simulink model "ProyectoControl"  (R2020b)
settings: Solver=VariableStepAuto  StartTime=0.0  StopTime=25  RelTol=1e-3
values from neighbouring files (symbols this model uses):
  A = [-0.0558 0.08 -0.997 0.0415 0.0033 ... (first row only)    [Control_proyecto.m]
  B = [0 0.00729 ... (first row only)    [Control_proyecto.m]
  C = [0 0 0 1 0 ... (first row only)    [Control_proyecto.m]
  D = [0 0;0 0]    [Control_proyecto.m]
  Ki = [Kaug(:,6) Kaug(:,7)]    [Control_proyecto.m]
  Kp = Kaug(:,1:5)    [Control_proyecto.m]
  lambda = 0.5    [Control_proyecto.m]
undefined symbols (not defined in the file or in its folder): DiscIntNeverNeededParam, L, sigbuilder_block
libraries: simulink_extras x10, simulink x3, eeGeneralControl x1
settings Model: Creator=agustin  LastModifiedBy=agustin

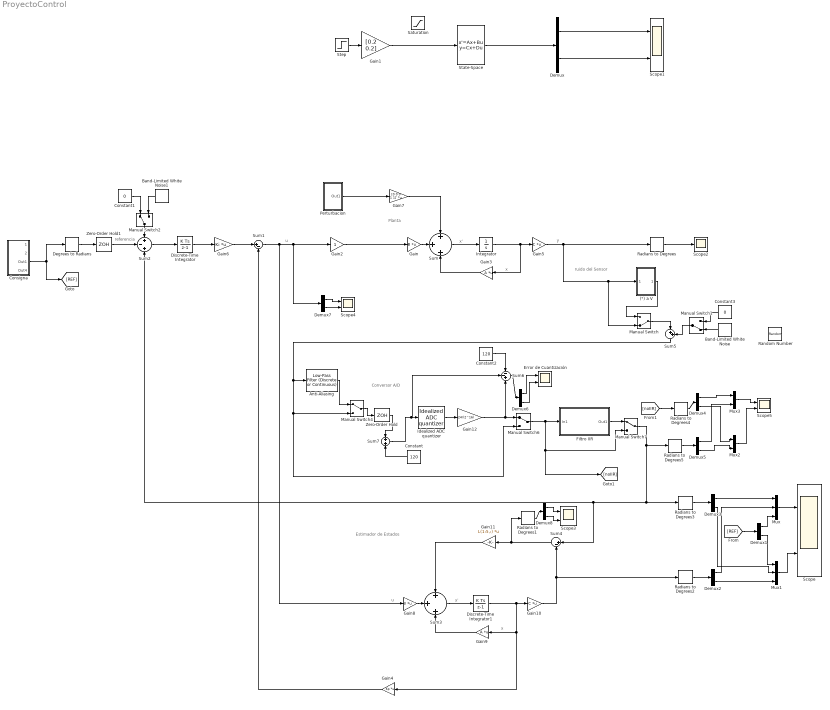
== system ProyectoControl ==
  note: Conversor A/D
  note: ruido del Sensor
  note: Estimador de Estados
  note: referencia
  note: Planta
  note: y
  note: x
  note: x'
  note: u
  note: x
  note: x'
  note: u
  (°) a V : Subsystem
  Anti-Aliasing : eeGeneralControl/Low-Pass Filter (Discrete or Continuous)  K=1  T=0.01  B=inf  A=-inf  init_option=Inherited from block input  x0=0  Ts=-1
  Band-Limited White Noise : simulink/Sources/Band-Limited White Noise  Cov=[70e-9]  Ts=0.1  seed=[23341]
  Band-Limited White Noise1 : simulink/Sources/Band-Limited White Noise  Cov=[0.25e-6]  Ts=0.1  seed=[23341]
  Consigna : Subsystem
  Constant : Constant  Value=120
  Constant1 : Constant  Value=0
  Constant2 : Constant  Value=120
  Constant3 : Constant  Value=0
  Degrees to Radians : simulink_extras/Transformations/Degrees to Radians
  Demux{,1..8} (9 alike) : Demux  Outputs=2
  Discrete-Time Integrator : DiscreteIntegrator  SampleTime=-1  ICPrevOutput=DiscIntNeverNeededParam  ICPrevScaledInput=DiscIntNeverNeededParam
  Discrete-Time Integrator1 : DiscreteIntegrator  SampleTime=-1  ICPrevOutput=DiscIntNeverNeededParam  ICPrevScaledInput=DiscIntNeverNeededParam
  Error de Cuantización : Scope  NumInputPorts=2
  Filtro IIR : Subsystem
  Gain : Gain  Gain=B  Multiplication=Matrix(K*u)
  Gain1 : Gain  Gain=[0.2 0.2]
  Gain10 : Gain  Gain=C  Multiplication=Matrix(K*u)
  Gain11 : Gain  Gain=L(1:5,:)  Multiplication=Matrix(K*u)
  Gain12 : Gain  Gain=24/(2^16)
  Gain2 : Gain
  Gain3 : Gain  Gain=A  Multiplication=Matrix(K*u)
  Gain4 : Gain  Gain=Kp  Multiplication=Matrix(K*u)
  Gain5 : Gain  Gain=C  Multiplication=Matrix(K*u)
  Gain6 : Gain  Gain=Ki  Multiplication=Matrix(K*u)
  Gain7 : Gain  Gain=[0 0 0 1 1]'  Multiplication=Matrix(K*u)
  Gain8 : Gain  Gain=B  Multiplication=Matrix(K*u)
  Gain9 : Gain  Gain=A  Multiplication=Matrix(K*u)
  Idealized ADC quantizer : simulink_extras/Additional Discrete/Idealized ADC quantizer  NumberOfConverterBits=16  Vmin=100  Vmax=140  OutputDataType=int32  OutputNegativeValues=on
  Integrator : Integrator
  Manual Switch : ManualSwitch  CurrentSetting=0
  Manual Switch1 : ManualSwitch  CurrentSetting=0
  Manual Switch{2,4,6..7} (4 alike) : ManualSwitch
  Mux : Mux  Inputs=3
  Mux1 : Mux  Inputs=3
  Mux2 : Mux  Inputs=2
  Mux3 : Mux  Inputs=2
  Perturbacion : Subsystem
  Radians to Degrees{,1..5} (6 alike) : simulink_extras/Transformations/Radians to Degrees
  Random Number : RandomNumber  Variance=70e-9  SampleTime=0.1
  Saturation : Saturate  UpperLimit=1  LowerLimit=-1
  Scope{,1,3..5} (5 alike) : Scope  NumInputPorts=2
  Scope2 : Scope
  State-Space : StateSpace  A=A  B=B  C=C  D=D  InitialCondition=0  ContinuousStateAttributes='position'
  Step : Step  SampleTime=0
  Sum : Sum  Inputs=+|+|+
  Sum1 : Sum  Inputs=|+-
  Sum2 : Sum  Inputs=+-+
  Sum3 : Sum  Inputs=+|+|+
  Sum4 : Sum  Inputs=|+-
  Sum5 : Sum  Inputs=|++
  Sum6 : Sum  Inputs=--+
  Sum7 : Sum
  Zero-Order Hold : ZeroOrderHold  SampleTime=1e-3
  Zero-Order Hold1 : ZeroOrderHold  SampleTime=1e-3
  wires:
  State-Space/1 -> Demux/1
  Step/1 -> Gain1/1
  Demux/1 -> Scope1/1
  Demux/2 -> Scope1/2
  Gain1/1 -> State-Space/1
  Gain/1 -> Sum/2
  Gain3/1 -> Sum/3
  Sum/1 -> Integrator/1
  Integrator/1 -> Gain3/1, Gain5/1
  Gain4/1 -> Sum1/2
  Gain6/1 -> Sum1/1
  Sum2/1 -> Discrete-Time Integrator/1
  Gain7/1 -> Sum/1
  Discrete-Time Integrator/1 -> Gain6/1
  Gain11/1 -> Sum3/1
  Gain8/1 -> Sum3/2
  Sum3/1 -> Discrete-Time Integrator1/1
  Gain9/1 -> Sum3/3
  Discrete-Time Integrator1/1 -> Gain4/1, Gain9/1, Gain10/1
  Sum1/1 -> Demux7/1, Gain2/1, Gain8/1
  Gain10/1 -> Sum4/2, Radians to Degrees2/1
  Sum4/1 -> Gain11/1, Radians to Degrees1/1
  Sum5/1 -> Anti-Aliasing/1, Manual Switch4/2, Manual Switch6/2
  Constant3/1 -> Manual Switch1/1
  Manual Switch1/1 -> Sum5/2
  Zero-Order Hold/1 -> Sum7/1
  Idealized ADC quantizer/1 -> Gain12/1
  Gain12/1 -> Sum6/3, Manual Switch6/1
  Filtro IIR/1(Out1) -> Manual Switch7/1
  Radians to Degrees1/1 -> Demux8/1
  Radians to Degrees2/1 -> Demux2/1
  Manual Switch4/1 -> Zero-Order Hold/1
  Anti-Aliasing/1 -> Manual Switch4/1
  Manual Switch6/1 -> Filtro IIR/1(In1), [noIIR], Manual Switch7/2
  Manual Switch7/1 -> Radians to Degrees5/1, Sum2/3, Sum4/1, Radians to Degrees3/1
  Zero-Order Hold1/1 -> Sum2/2
  Degrees to Radians/1 -> Zero-Order Hold1/1
  [REF] -> Demux1/1
  Perturbacion/1(Out1) -> Gain7/1
  Band-Limited White Noise1/1 -> Manual Switch2/2
  Constant1/1 -> Manual Switch2/1
  Manual Switch2/1 -> Sum2/1
  Consigna/3(Out1) -> [REF], Degrees to Radians/1
  Mux/1 -> Scope/1
  Mux1/1 -> Scope/2
  Radians to Degrees3/1 -> Demux3/1
  Demux2/2 -> Mux1/3
  Demux2/1 -> Mux/2
  Demux3/2 -> Mux1/2
  Demux1/2 -> Mux1/1
  Demux3/1 -> Mux/1
  Demux1/1 -> Mux/3
  [noIIR] -> Radians to Degrees4/1
  Mux3/1 -> Scope5/1
  Mux2/1 -> Scope5/2
  Demux4/1 -> Mux3/1
  Demux5/1 -> Mux3/2
  Demux4/2 -> Mux2/1
  Demux5/2 -> Mux2/2
  Radians to Degrees4/1 -> Demux4/1
  Radians to Degrees5/1 -> Demux5/1
  Sum6/1 -> Demux6/1
  Demux6/1 -> Error de Cuantización/1
  Demux6/2 -> Error de Cuantización/2
  Demux7/1 -> Scope4/1
  Demux7/2 -> Scope4/2
  Gain2/1 -> Gain/1
  Demux8/1 -> Scope3/1
  Demux8/2 -> Scope3/2
  Band-Limited White Noise/1 -> Manual Switch1/2
  Constant/1 -> Sum7/2
  Sum7/1 -> Sum6/2, Idealized ADC quantizer/1
  Constant2/1 -> Sum6/1
  Gain5/1 -> Radians to Degrees/1, Manual Switch/2, (°) a V/1(In1)
  Radians to Degrees/1 -> Scope2/1
  (°) a V/1(Out1) -> Manual Switch/1
  Manual Switch/1 -> Sum5/1

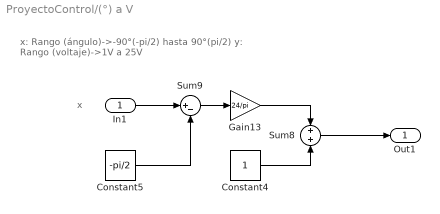
== system ProyectoControl/(°) a V ==
  note: x
  note: x: Rango (ángulo)->-90°(-pi/2) hasta 90°(pi/2)
      | y: Rango (voltaje)->1V a 25V
  In1 : Inport
  Constant4 : Constant
  Constant5 : Constant  Value=-pi/2
  Gain13 : Gain  Gain=24/pi
  Sum8 : Sum
  Sum9 : Sum  Inputs=|+-
  Out1 : Outport
  wires:
  In1/1 -> Sum9/1
  Constant5/1 -> Sum9/2
  Sum9/1 -> Gain13/1
  Sum8/1 -> Out1/1
  Gain13/1 -> Sum8/1
  Constant4/1 -> Sum8/2

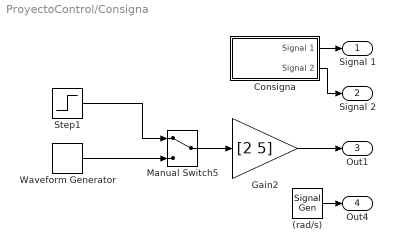
== system ProyectoControl/Consigna ==
  "(rad/s) " : SignalGenerator  WaveForm=square  Amplitude=0.2  Frequency=0.1  Units=rad/sec
  Consigna : Subsystem  Tag=STV Subsys  LoadFcn=sigbuilder_block('load');  StartFcn=sigbuilder_block('start');  StopFcn=sigbuilder_block('stop');  ClipboardFcn=sigbuilder_block('clipboard');  mask(Sigbuilder block){tuvar=[0:10]}
      mask help: Simulink:masks:SigbuilderBlock_MD
      mask init:
      | if ~strcmp(get_param(bdroot(gcbh),'SimulationStatus'),'stopped') tuvar = sigbuilder_block('maskInit'); end
      settings: CopyFcn=sigbuilder_block('copy');  DeleteFcn=sigbuilder_block('delete');  ModelCloseFcn=sigbuilder_block('modelClose');  PreSaveFcn=sigbuilder_block('preSave');  PauseFcn=sigbuilder_block('pause');  ContinueFcn=sigbuilder_block('continue');  NameChangeFcn=sigbuilder_block('namechange');  OpenFcn=sigbuilder_block('open',[311.25 87.75 550.5 359.25 ]);  CloseFcn=sigbuilder_block('close');
      mask Display: plot(0, 0, 100, 100,[2, 2, 32, 32, 2], [68, 8, 8, 68, 68],[32, 2], [38, 38], [32, 19, 2],[53, 60, 44], [32, 17, 17, 2],[16, 16, 31, 31]);txt = getActiveGroup(gcbh);text(2, 100, txt,'verticalAlignment', 'top');
  Gain2 : Gain  Gain=[2 5]
  Manual Switch5 : ManualSwitch
  Step1 : Step  SampleTime=0
  Waveform Generator : simulink/Sources/Waveform Generator  OutMin=[]  OutMax=[]  OutDataTypeStr=double  SelectedSignal=1  Signals=sin('Amplitude', 1, 'Frequency', 0.1, 'Phase', 0)  BlockNames=MultiportSwitch_92f0ff05a9a94f3  SampleTime=0.1
  Signal 1 : Outport
  Signal 2 : Outport  Port=2
  Out1 : Outport  Port=3
  Out4 : Outport  Port=4
  wires:
  Gain2/1 -> Out1/1
  Manual Switch5/1 -> Gain2/1
  Step1/1 -> Manual Switch5/1
  Waveform Generator/1 -> Manual Switch5/2
  "(rad/s) "/1 -> Out4/1
  Consigna/1(Signal 1) -> Signal 1/1
  Consigna/2(Signal 2) -> Signal 2/1

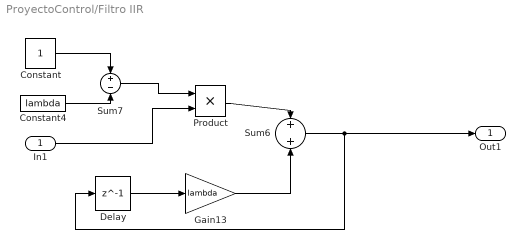
== system ProyectoControl/Filtro IIR ==
  In1 : Inport
  Constant : Constant
  Constant4 : Constant  Value=lambda
  Delay : Delay  DelayLength=1  InitialCondition=0
  Gain13 : Gain  Gain=lambda
  Product : Product
  Sum6 : Sum
  Sum7 : Sum  Inputs=+-
  Out1 : Outport
  wires:
  Product/1 -> Sum6/1
  Delay/1 -> Gain13/1
  In1/1 -> Product/2
  Sum6/1 -> Out1/1, Delay/1
  Sum7/1 -> Product/1
  Gain13/1 -> Sum6/2
  Constant/1 -> Sum7/1
  Constant4/1 -> Sum7/2

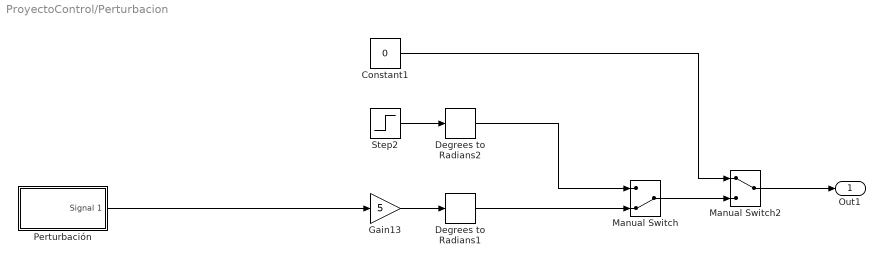
== system ProyectoControl/Perturbacion ==
  Constant1 : Constant  Value=0
  Degrees to Radians1 : simulink_extras/Transformations/Degrees to Radians
  Degrees to Radians2 : simulink_extras/Transformations/Degrees to Radians
  Gain13 : Gain  Gain=5
  Manual Switch : ManualSwitch  CurrentSetting=0
  Manual Switch2 : ManualSwitch
  Perturbación : Subsystem  Tag=STV Subsys  LoadFcn=sigbuilder_block('load');  StartFcn=sigbuilder_block('start');  StopFcn=sigbuilder_block('stop');  ClipboardFcn=sigbuilder_block('clipboard');  mask(Sigbuilder block){tuvar=[0:10]}
      mask help: Simulink:masks:SigbuilderBlock_MD
      mask init:
      | if ~strcmp(get_param(bdroot(gcbh),'SimulationStatus'),'stopped') tuvar = sigbuilder_block('maskInit'); end
      settings: CopyFcn=sigbuilder_block('copy');  DeleteFcn=sigbuilder_block('delete');  ModelCloseFcn=sigbuilder_block('modelClose');  PreSaveFcn=sigbuilder_block('preSave');  PauseFcn=sigbuilder_block('pause');  ContinueFcn=sigbuilder_block('continue');  NameChangeFcn=sigbuilder_block('namechange');  OpenFcn=sigbuilder_block('open',[437.6 153 550.4 359.25 ]);  CloseFcn=sigbuilder_block('close');
      mask Display: plot(0, 0, 100, 100,[2, 2, 32, 32, 2], [68, 8, 8, 68, 68],[32, 2], [38, 38], [32, 19, 2],[53, 60, 44], [32, 17, 17, 2],[16, 16, 31, 31]);txt = getActiveGroup(gcbh);text(2, 100, txt,'verticalAlignment', 'top');
  Step2 : Step  After=2  SampleTime=0
  Out1 : Outport
  wires:
  Degrees to Radians1/1 -> Manual Switch/2
  Manual Switch/1 -> Manual Switch2/2
  Constant1/1 -> Manual Switch2/1
  Manual Switch2/1 -> Out1/1
  Perturbación/1(Signal 1) -> Gain13/1
  Step2/1 -> Degrees to Radians2/1
  Gain13/1 -> Degrees to Radians1/1
  Degrees to Radians2/1 -> Manual Switch/1

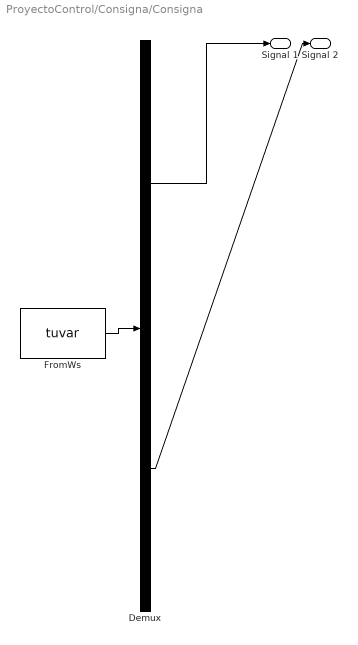
== system ProyectoControl/Consigna/Consigna ==
  Demux : Demux  Tag=STV Demux  Outputs=2
      settings: DisplayOption=none
  FromWs : FromWorkspace  Tag=STV FromWs  VariableName=tuvar
      SigBuilderData=|
      | common.afterFinalStr = 'Extrapolate'
      | common.sampleTime = 0
      | dataSet.timeRange = [0 10]
      | dataSet.name = 'Group 1'
      | sbobj.Groups.Name = 'Group 1'
      | sbobj.Groups.Signals(1).Name = 'Signal 1'
      | sbobj.Groups.Signals(1).XData = [0 2 4.5 5.5 8 9.02 9.02 10]
      | sbobj.Groups.Signals(1).YData = [0 0 1 1 -1 -1 0 0]
      | sbobj.Groups.Signals(2).Name = 'Signal 2'
      | sbobj.Groups.Signals(2).XData = [0 2 4 6 8 10]
      | sbobj.Groups.Signals(2).YData = [0 0 1 1 0 0]
  Signal 1 : Outport  Tag=STV Outport
  Signal 2 : Outport  Tag=STV Outport  Port=2
  wires:
  Demux/1 -> Signal 1/1
  FromWs/1 -> Demux/1
  Demux/2 -> Signal 2/1

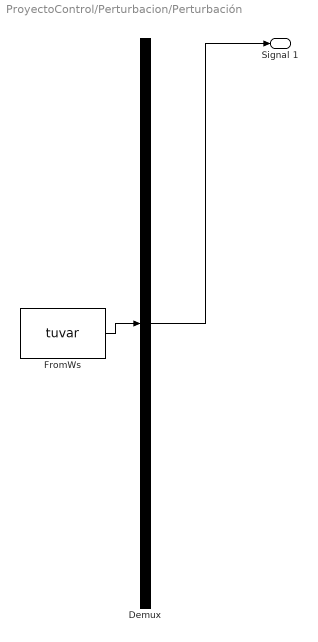
== system ProyectoControl/Perturbacion/Perturbación ==
  Demux : Demux  Tag=STV Demux  Outputs=1
      settings: DisplayOption=none
  FromWs : FromWorkspace  Tag=STV FromWs  VariableName=tuvar
      SigBuilderData=|
      | common.afterFinalStr = 'Extrapolate'
      | common.sampleTime = 0
      | dataSet.timeRange = [0 10]
      | dataSet.name = 'Group 1'
      | sbobj.Groups.Name = 'Group 1'
      | sbobj.Groups.Signals.Name = 'Signal 1'
      | sbobj.Groups.Signals.XData = [0 4 4.5 5.5 6 10]
      | sbobj.Groups.Signals.YData = [0 0 1 1 0 0]
  Signal 1 : Outport  Tag=STV Outport
  wires:
  Demux/1 -> Signal 1/1
  FromWs/1 -> Demux/1
